simulink model "Motor_new"  (Simulink 7.1)
settings: Solver=ode45  StartTime=0.0  StopTime=1  MaxStep=0.0001  RelTol=1e-3
undefined symbols (not defined in the file): amplitude, duty_cycle, Jm, on_time, pwm_periode, resolution
libraries: simulink x1
settings Model: Creator=dep19025415  LastModifiedBy=dep19025415

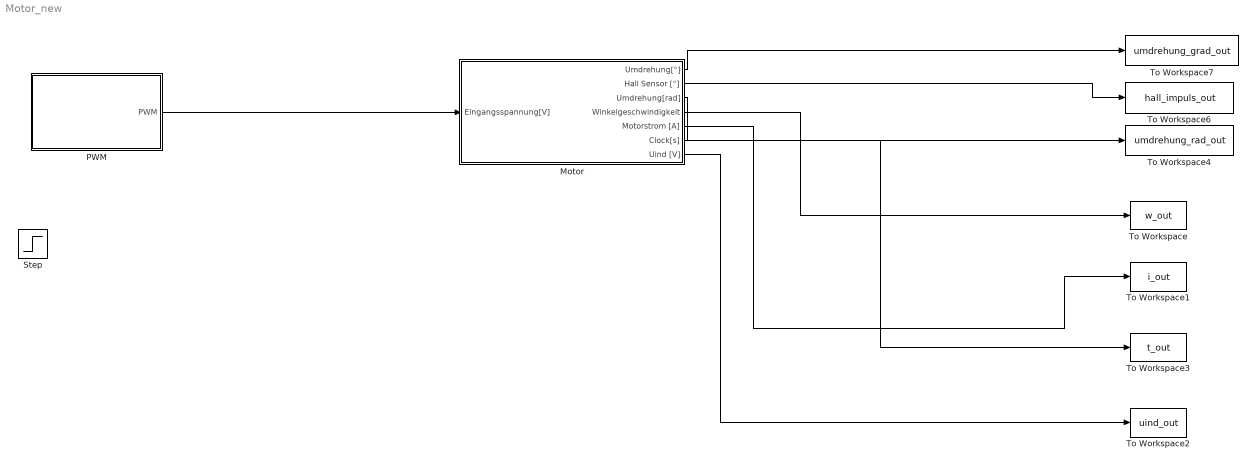
== system Motor_new ==
  Motor : Subsystem
  PWM : Subsystem  mask{ontime=on_time, amp=amplitude, duty=duty_cycle, tpwm=pwm_periode, max=resolution}
      mask prompts: ontime "On time (s)"; amp "Amplitude (V)"; duty "Duty cycle (%)"; tpwm "PWM period (s)"; max "Resolution"
  Step : Step  Time=10e-3  Before=8  After=0  SampleTime=0
  To Workspace : ToWorkspace  VariableName=w_out  SampleTime=-1  SaveFormat=Structure
  To Workspace1 : ToWorkspace  VariableName=i_out  SampleTime=-1  SaveFormat=Structure
  To Workspace2 : ToWorkspace  VariableName=uind_out  SampleTime=-1  SaveFormat=Structure
  To Workspace3 : ToWorkspace  VariableName=t_out  SampleTime=-1  SaveFormat=Structure
  To Workspace4 : ToWorkspace  VariableName=umdrehung_rad_out  SampleTime=-1  SaveFormat=Structure
  To Workspace6 : ToWorkspace  VariableName=hall_impuls_out  SampleTime=-1  SaveFormat=Structure
  To Workspace7 : ToWorkspace  VariableName=umdrehung_grad_out  SampleTime=-1  SaveFormat=Structure
  wires:
  Motor/6(Clock[s]) -> To Workspace3/1
  Motor/2(Hall Sensor [°]) -> To Workspace6/1
  Motor/1(Umdrehung[°]) -> To Workspace7/1
  Motor/3(Umdrehung[rad]) -> To Workspace4/1
  Motor/4(Winkelgeschwindigkeit) -> To Workspace/1
  Motor/5(Motorstrom [A]) -> To Workspace1/1
  Motor/7(Uind [V]) -> To Workspace2/1
  PWM/1(PWM) -> Motor/1(Eingangsspannung[V])

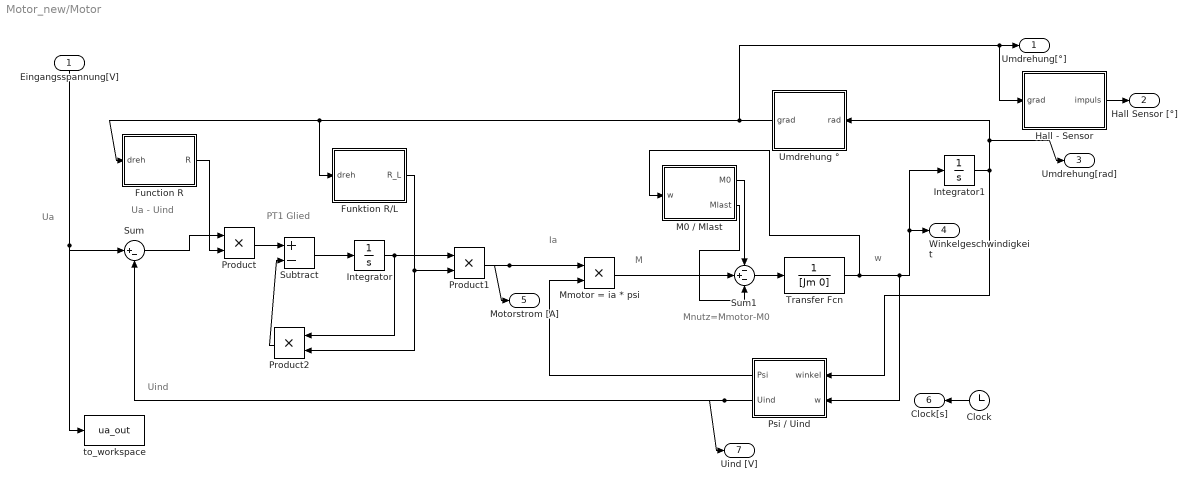
== system Motor_new/Motor ==
  note: PT1 Glied
  note: M
  note: Ua - Uind
  note: Uind
  note: Ua
  note: Mnutz=Mmotor-M0
  note: Ia
  note: w
  Eingangsspannung[V] : Inport  Orientation=down
  Clock : Clock
      settings: Decimation=10
  Function R : Stateflow chart
  Funktion R/L : Stateflow chart
  Hall - Sensor : Stateflow chart
  Integrator : Integrator
  Integrator1 : Integrator
  M0 / Mlast : Stateflow chart
  Mmotor = ia * psi : Product  OutDataType=sfix(16)  OutScaling=2^0  RndMeth=Zero
  Product : Product  OutDataType=sfix(16)  OutScaling=2^0  RndMeth=Zero
  Product1 : Product  OutDataType=sfix(16)  OutScaling=2^0  RndMeth=Zero
  Product2 : Product  Orientation=left  OutDataType=sfix(16)  OutScaling=2^0  RndMeth=Zero
  Psi / Uind : Stateflow chart  Orientation=left
  Subtract : Sum  Inputs=+-  OutDataType=sfix(16)  OutScaling=2^-10
  Sum : Sum  Inputs=|+-  OutDataType=sfix(16)  OutScaling=2^0
  Sum1 : Sum  Inputs=-+-  OutDataType=sfix(16)  OutScaling=2^0
  Transfer Fcn : TransferFcn  Denominator=[Jm 0]
  Umdrehung ° : Stateflow chart  Orientation=left
  to_workspace : ToWorkspace  VariableName=ua_out  SampleTime=-1  SaveFormat=Structure
  Umdrehung[°] : Outport
  Hall Sensor [°] : Outport  Port=2
  Umdrehung[rad] : Outport  Port=3
  Winkelgeschwindigkeit : Outport  Port=4
  Motorstrom [A] : Outport  Port=5
  Clock[s] : Outport  Orientation=left  Port=6
  Uind [V] : Outport  Port=7
  wires:
  Product1/1 -> Mmotor = ia * psi/1, Motorstrom [A]/1
  Sum/1 -> Product/1
  Umdrehung °/1(grad) -> Funktion R/L/1(dreh), Function R/1(dreh), Hall - Sensor/1(grad), Umdrehung[°]/1
  Psi / Uind/2(Uind) -> Sum/2, Uind [V]/1
  Psi / Uind/1(Psi) -> Mmotor = ia * psi/2
  Mmotor = ia * psi/1 -> Sum1/2
  Integrator1/1 -> Umdrehung °/1(rad), Umdrehung[rad]/1, Psi / Uind/1(winkel)
  Transfer Fcn/1 -> Integrator1/1, Winkelgeschwindigkeit/1, Psi / Uind/2(w), M0 / Mlast/1(w)
  Sum1/1 -> Transfer Fcn/1
  Funktion R/L/1(R_L) -> Product1/2, Product2/2
  Function R/1(R) -> Product/2
  Product2/1 -> Subtract/2
  Integrator/1 -> Product1/1, Product2/1
  Subtract/1 -> Integrator/1
  Product/1 -> Subtract/1
  Eingangsspannung[V]/1 -> to_workspace/1, Sum/1
  M0 / Mlast/2(Mlast) -> Sum1/3
  M0 / Mlast/1(M0) -> Sum1/1
  Hall - Sensor/1(impuls) -> Hall Sensor [°]/1
  Clock/1 -> Clock[s]/1

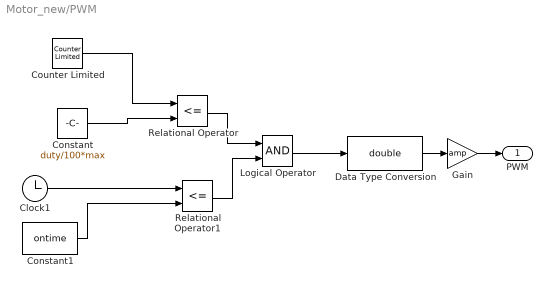
== system Motor_new/PWM ==
  Clock1 : Clock
      settings: Decimation=10
  Constant : Constant  Value=duty/100*max  OutDataType=sfix(16)  OutScaling=2^0
  Constant1 : Constant  Value=ontime  OutDataType=sfix(16)  OutScaling=2^0
  Counter Limited : simulink/Sources/Counter Limited  SystemSampleTime=-1  uplimit=max  tsamp=tpwm/max
  Data Type Conversion : DataTypeConversion  OutDataTypeMode=double  OutDataType=sfix(16)  OutScaling=2^0  OutDataTypeStr=double
  Gain : Gain  Gain=amp  ParameterDataType=sfix(16)  ParameterScaling=2^0  OutDataType=sfix(16)  OutScaling=2^0
  Logical Operator : Logic  AllPortsSameDT=off  OutDataTypeMode=boolean  OutDataTypeStr=boolean
  Relational Operator : RelationalOperator  Operator=<=  LogicOutDataTypeMode=boolean  OutDataTypeStr=boolean
  Relational Operator1 : RelationalOperator  Operator=<=  LogicOutDataTypeMode=boolean  OutDataTypeStr=boolean
  PWM : Outport
  wires:
  Counter Limited/1 -> Relational Operator/1
  Constant/1 -> Relational Operator/2
  Clock1/1 -> Relational Operator1/1
  Constant1/1 -> Relational Operator1/2
  Relational Operator/1 -> Logical Operator/1
  Relational Operator1/1 -> Logical Operator/2
  Logical Operator/1 -> Data Type Conversion/1
  Data Type Conversion/1 -> Gain/1
  Gain/1 -> PWM/1

== matlab function Motor/M0 / Mlast ==
  data: w input double; M0 output double; Mlast output double
function [M0,Mlast] = fcn(w)
% Um zu verhindern, dass die Simulation bei einer Versorgungsspannung von 0V
% den Motor Rückwärts laufen lässt, werden die Reibungsverluste erst ab einem
% sich drehenden Motor berücksichtigt.


M0=0;
Mlast=0;

if w > 0
    M0=0.559e-3;
     Mlast=5.7e-3;
end
end

== matlab function Motor/Umdrehung ° ==
  data: rad input double; grad output double
function grad = fcn(rad)
% In dieser Funktion werden die Umdrehung die der Motor sich dreht [in Grad]
% so umgerechnet, dass als Ausgang immer nur Umdrehungen von 0-360° angezeigt
% werden


a = (rad*180/pi)/360;
b = fix(a);
c = a - b;
grad = c * 360;

end

== matlab function Motor/Function R ==
  data: dreh input double; R output double
function R = fcn(dreh)
% In dieser Funktion wird abhängig vom Drehwinkel des Motors der Widerstandswert für R geändert.
% Schließt der Schleifkontakt zwei Kommutierungen kurz, so verringer sich der Widerstand der 
% Drahtwindungen, da eine Spule kurzgeschlossen wird.

R = (1/6.6);
% if (dreh >= 60 && dreh <=60.2) || (dreh >= 120 && dreh <= 120.2) || (dreh >= 180 && dreh <= 180.2) || (dreh >= 240 && dreh <= 240.2) || (dreh >= 300 && dreh <= 300.2) || (dreh >= 0 && dreh <= 0.2)
%    R = (1/5); 
% end

end

== matlab function Motor/Funktion R/L ==
  data: dreh input double; R_L output double
function R_L = fcn(dreh)
% In dieser Funktion wird abhängig vom Drehwinkel des Motors der Wert für R und L geändert.
% Schließt der Schleifkontakt zwei Kommutierungen kurz, so verringer sich der Widerstand, als 
% als auch die Induktivität der Spulen, da eine Spule kurzgeschlossen wird. 


R_L = (6/7.3e-3);
% if (dreh >= 60 && dreh <=60.2) || (dreh >= 120 && dreh <= 120.2) || (dreh >= 180 && dreh <= 180.2) || (dreh >= 240 && dreh <= 240.2) || (dreh >= 300 && dreh <= 300.2) || (dreh >= 0 && dreh <= 0.2)
%     R_L = (5/5.5e-3); 
% end

end

== matlab function Motor/Psi / Uind ==
  data: winkel input double; w input double; Psi output double; Uind output double
function [Psi, Uind] = fcn(winkel, w)
% In dieser Funktion wird abhängig von der Drehposition des Motors
% die induzierte Spannung (Uind) als auch der magnetische Verkettete
% Fluss (Psi) berechnet

Uind = nan;
EMF = 5;
psicon = EMF / (100 * pi);
%Uind = 2 * pi / 6 * w * psicon * (sin(w*t+pi/3*(1-fix(3/pi*w*t))));
Psi =  psicon * (sin(winkel+pi/3*(1-fix(3/pi*winkel))));
Uind = (2 * pi / 6) * w * psicon * (sin(winkel+pi/3*(1-fix(3/pi*winkel))));;


% if t <= 0
%     Uind = 0;
% end
% if t<=0 
%     Uind=0;
% end


end

== matlab function Motor/Hall - Sensor ==
  data: grad input double; impuls output double
function impuls = fcn(grad)
% In dieser Funktion werden die Umdrehung die der Motor sich dreht [in Grad]
% so umgerechnet, dass als Ausgang immer nur Umdrehungen von 0-360° angezeigt
% werden


impuls = 0;
if (grad >=22.5 && grad <= 22.6)
    impuls = 1;
end
if (grad >=45 && grad <= 45.1)
    impuls = 1;
end
if (grad >=67.5 && grad <= 67.6)
    impuls = 1;
end
if (grad >=90 && grad <= 90.1)
    impuls = 1;
end
if (grad >=112.5 && grad <= 112.6)
    impuls = 1;
end
if (grad >=135 && grad <= 135.1)
    impuls = 1;
end
if (grad >=157.5 && grad <= 157.6)
    impuls = 1;
end
if (grad >=180 && grad <= 180.1)
    impuls = 1;
end
if (grad >=202.5 && grad <= 202.6)
    impuls = 1;
end
if (grad >=225 && grad <= 225.1)
    impuls = 1;
end
if (grad >=247.5 && grad <= 247.6)
    impuls = 1;
end
if (grad >=270 && grad <= 270.1)
    impuls = 1;
end
if (grad >=292.5 && grad <= 292.6)
    impuls = 1;
end
if (grad >=315 && grad <= 315.1)
    impuls = 1;
end
if (grad >=337.5 && grad <= 337.6)
    impuls = 1;
end
if (grad >=0 && grad <= 0.1)
    impuls = 1;
end

end
